simulink model "System_Identification_Parametric"  (R2019a)
settings: Solver=FixedStepAuto  StartTime=0.0  StopTime=1  FixedStep=1e-3  RelTol=1e-3
libraries: simulink x1, cstblocks x1
settings Model: Creator=capn  LastModifiedBy=emma
settings DataIOCC: ReturnWorkspaceOutputs=off
settings DebuggingCC: ArithmeticOperatorsInVariantConditions=warning
settings SFSimCC: SimUseLocalCustomCode=off
settings RTWCC: RTWUseLocalCustomCode=off
settings CodeAppCC: StateflowObjectComments=on

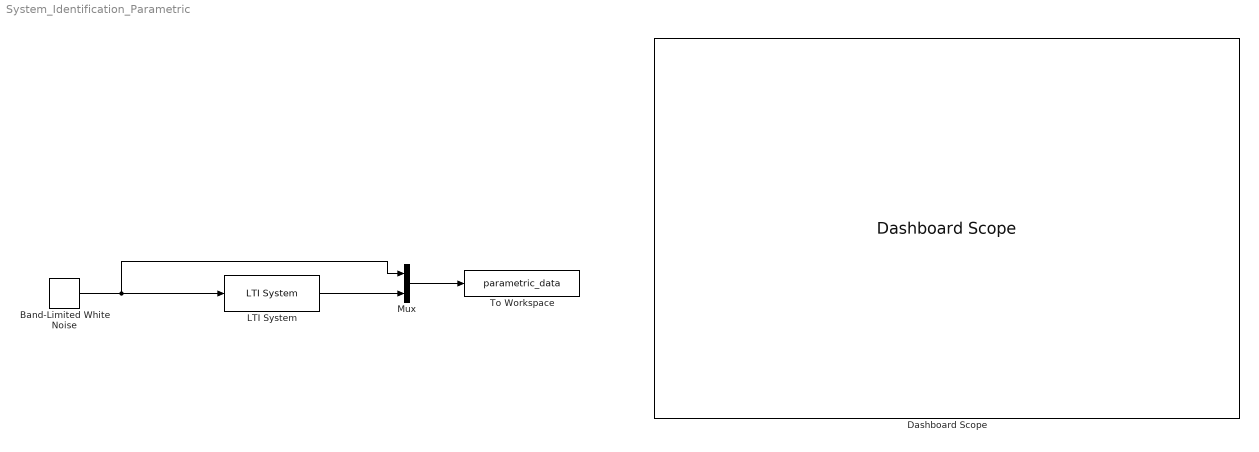
== system System_Identification_Parametric ==
  Band-Limited White Noise : simulink/Sources/Band-Limited White Noise  Cov=[0.1]  Ts=0.01  seed=[23341]
  Dashboard Scope : DashboardScope
  LTI System : cstblocks/LTI System  sys=tf(1,[1 1 5])  IC=[]
  Mux : Mux  Inputs=2
  To Workspace : ToWorkspace  VariableName=parametric_data  SampleTime=-1
  wires:
  Band-Limited White Noise/1 -> LTI System/1, Mux/1
  LTI System/1 -> Mux/2
  Mux/1 -> To Workspace/1
